simulink model "skarab_adc4x3g14_byp"  (R2018a)
settings: Solver=VariableStepAuto  StartTime=0.0  StopTime=10.0  RelTol=1e-3
libraries: xbsIndex_r4 x113
settings Model: Creator=aisaacson  LastModifiedBy=aisaacson

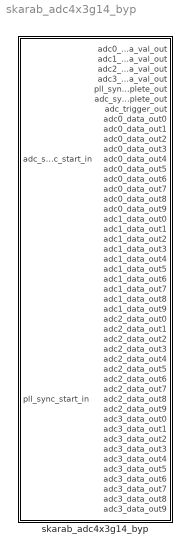
== system skarab_adc4x3g14_byp ==
  skarab_adc4x3g14_byp : Subsystem  Tag=xps:skarab_adc4x3g_14_byp  mask(hmc){mez=2}
      mask prompts: mez "Mezzanine slot"
      mask help: Interface to ADC cards available on SKARAB boards.
      mask init:
      | skarab_adc4x3g14_byp_mask(gcb);
      mask TypeOptions mez: 0 | 1 | 2 | 3
      mask DialogControl Container6 Prompt: Parameters

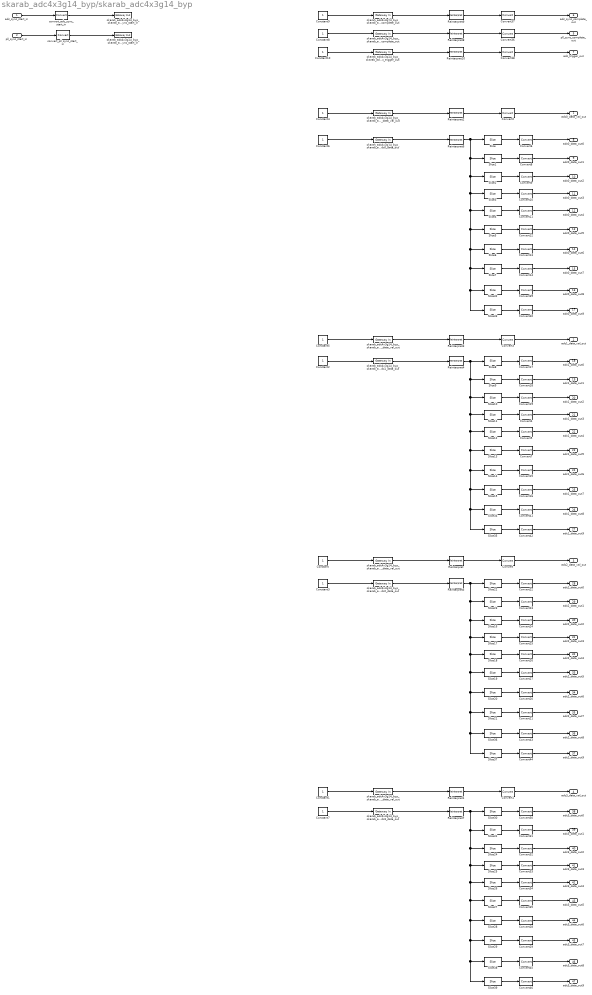
== system skarab_adc4x3g14_byp/skarab_adc4x3g14_byp ==
  adc_sync_start_in : Inport
  pll_sync_start_in : Inport  Port=2
  Constant{,1..10} (11 alike) : Constant
  Convert{,1..3,36..38} (7 alike) : xbsIndex_r4/Convert  gui_display_data_type=Boolean  arith_type=Boolean  n_bits=16  bin_pt=14  float_type=Single  exp_bits=8  fraction_bits=24  quantization=Truncate  overflow=Wrap  en=off  latency=0  pipeline=off  dbl_ovrd=off  block_type=convert
  Convert{4..35,39..46} (40 alike) : xbsIndex_r4/Convert  gui_display_data_type=Fixed-point  arith_type="Signed  (2's comp)"  n_bits=12  bin_pt=0  float_type=Single  exp_bits=8  fraction_bits=24  quantization=Truncate  overflow=Wrap  en=off  latency=0  pipeline=off  dbl_ovrd=off  block_type=convert
  Reinterpret{,1..10} (11 alike) : xbsIndex_r4/Reinterpret  force_arith_type=on  arith_type=Unsigned  force_bin_pt=on  bin_pt=0  block_type=reinterpret
  Slice{,8,22,30} (4 alike) : xbsIndex_r4/Slice  nbits=12  boolean_output=off  mode=Lower Bit Location + Width  bit1=0  base1=MSB of Input  bit0=0  base0=LSB of Input  dbl_ovrd=off  block_type=slice
  Slice{1,9,23,31} (4 alike) : xbsIndex_r4/Slice  nbits=12  boolean_output=off  mode=Lower Bit Location + Width  bit1=0  base1=MSB of Input  bit0=12  base0=LSB of Input  dbl_ovrd=off  block_type=slice
  Slice{2,10,16,24} (4 alike) : xbsIndex_r4/Slice  nbits=12  boolean_output=off  mode=Lower Bit Location + Width  bit1=0  base1=MSB of Input  bit0=24  base0=LSB of Input  dbl_ovrd=off  block_type=slice
  Slice{3,11,17,25} (4 alike) : xbsIndex_r4/Slice  nbits=12  boolean_output=off  mode=Lower Bit Location + Width  bit1=0  base1=MSB of Input  bit0=36  base0=LSB of Input  dbl_ovrd=off  block_type=slice
  Slice{4,12,18,26} (4 alike) : xbsIndex_r4/Slice  nbits=12  boolean_output=off  mode=Lower Bit Location + Width  bit1=0  base1=MSB of Input  bit0=48  base0=LSB of Input  dbl_ovrd=off  block_type=slice
  Slice{5,13,19,27} (4 alike) : xbsIndex_r4/Slice  nbits=12  boolean_output=off  mode=Lower Bit Location + Width  bit1=0  base1=MSB of Input  bit0=60  base0=LSB of Input  dbl_ovrd=off  block_type=slice
  Slice{6,14,20,28} (4 alike) : xbsIndex_r4/Slice  nbits=12  boolean_output=off  mode=Lower Bit Location + Width  bit1=0  base1=MSB of Input  bit0=72  base0=LSB of Input  dbl_ovrd=off  block_type=slice
  Slice{7,15,21,29} (4 alike) : xbsIndex_r4/Slice  nbits=12  boolean_output=off  mode=Lower Bit Location + Width  bit1=0  base1=MSB of Input  bit0=84  base0=LSB of Input  dbl_ovrd=off  block_type=slice
  Slice{32,34,36,38} (4 alike) : xbsIndex_r4/Slice  nbits=12  boolean_output=off  mode=Lower Bit Location + Width  bit1=0  base1=MSB of Input  bit0=96  base0=LSB of Input  dbl_ovrd=off  block_type=slice
  Slice{33,35,37,39} (4 alike) : xbsIndex_r4/Slice  nbits=12  boolean_output=off  mode=Lower Bit Location + Width  bit1=0  base1=MSB of Input  bit0=108  base0=LSB of Input  dbl_ovrd=off  block_type=slice
  convert_adc_sync_start_in : xbsIndex_r4/Convert  gui_display_data_type=Boolean  arith_type=Boolean  n_bits=16  bin_pt=14  float_type=Single  exp_bits=8  fraction_bits=24  quantization=Truncate  overflow=Wrap  en=off  latency=0  pipeline=off  dbl_ovrd=off  block_type=convert
  convert_pll_sync_start_in : xbsIndex_r4/Convert  gui_display_data_type=Boolean  arith_type=Boolean  n_bits=16  bin_pt=14  float_type=Single  exp_bits=8  fraction_bits=24  quantization=Truncate  overflow=Wrap  en=off  latency=0  pipeline=off  dbl_ovrd=off  block_type=convert
  skarab_adc4x3g14_byp_skarab_adc4x3g14_byp_adc0_data_out : xbsIndex_r4/Gateway In  gui_display_data_type=Fixed-point  arith_type=Unsigned  n_bits=128  bin_pt=0  preci_type=Single  exp_width=8  frac_width=24  rows=1  columns=1  quantization=Truncate  overflow=Wrap  period=1  UseAsADC=off  ADCChannel='1'  interface=None  automatic_assignment=on  address_offset=hex2dec('00')  intf_name=''  intf_description=''  default_value=0  timing_constraint=None  locs_specified=off  LOCs={}  io_standard={}  inherit_from_input=off  hdl_port=on  dbl_ovrd=off  block_type=gatewayin
  skarab_adc4x3g14_byp_skarab_adc4x3g14_byp_adc0_data_val_out : xbsIndex_r4/Gateway In  gui_display_data_type=Boolean  arith_type=Boolean  n_bits=16  bin_pt=14  preci_type=Single  exp_width=8  frac_width=24  rows=1  columns=1  quantization="Round  (unbiased: +/- Inf)"  overflow=Saturate  period=1  UseAsADC=off  ADCChannel='1'  interface=None  automatic_assignment=on  address_offset=hex2dec('00')  intf_name=''  intf_description=''  default_value=0  timing_constraint=None  locs_specified=off  LOCs={}  io_standard={}  inherit_from_input=off  hdl_port=on  dbl_ovrd=off  block_type=gatewayin
  skarab_adc4x3g14_byp_skarab_adc4x3g14_byp_adc1_data_out : xbsIndex_r4/Gateway In  gui_display_data_type=Fixed-point  arith_type=Unsigned  n_bits=128  bin_pt=0  preci_type=Single  exp_width=8  frac_width=24  rows=1  columns=1  quantization=Truncate  overflow=Wrap  period=1  UseAsADC=off  ADCChannel='1'  interface=None  automatic_assignment=on  address_offset=hex2dec('00')  intf_name=''  intf_description=''  default_value=0  timing_constraint=None  locs_specified=off  LOCs={}  io_standard={}  inherit_from_input=off  hdl_port=on  dbl_ovrd=off  block_type=gatewayin
  skarab_adc4x3g14_byp_skarab_adc4x3g14_byp_adc1_data_val_out : xbsIndex_r4/Gateway In  gui_display_data_type=Boolean  arith_type=Boolean  n_bits=16  bin_pt=14  preci_type=Single  exp_width=8  frac_width=24  rows=1  columns=1  quantization="Round  (unbiased: +/- Inf)"  overflow=Saturate  period=1  UseAsADC=off  ADCChannel='1'  interface=None  automatic_assignment=on  address_offset=hex2dec('00')  intf_name=''  intf_description=''  default_value=0  timing_constraint=None  locs_specified=off  LOCs={}  io_standard={}  inherit_from_input=off  hdl_port=on  dbl_ovrd=off  block_type=gatewayin
  skarab_adc4x3g14_byp_skarab_adc4x3g14_byp_adc2_data_out : xbsIndex_r4/Gateway In  gui_display_data_type=Fixed-point  arith_type=Unsigned  n_bits=128  bin_pt=0  preci_type=Single  exp_width=8  frac_width=24  rows=1  columns=1  quantization=Truncate  overflow=Wrap  period=1  UseAsADC=off  ADCChannel='1'  interface=None  automatic_assignment=on  address_offset=hex2dec('00')  intf_name=''  intf_description=''  default_value=0  timing_constraint=None  locs_specified=off  LOCs={}  io_standard={}  inherit_from_input=off  hdl_port=on  dbl_ovrd=off  block_type=gatewayin
  skarab_adc4x3g14_byp_skarab_adc4x3g14_byp_adc2_data_val_out : xbsIndex_r4/Gateway In  gui_display_data_type=Boolean  arith_type=Boolean  n_bits=16  bin_pt=14  preci_type=Single  exp_width=8  frac_width=24  rows=1  columns=1  quantization="Round  (unbiased: +/- Inf)"  overflow=Saturate  period=1  UseAsADC=off  ADCChannel='1'  interface=None  automatic_assignment=on  address_offset=hex2dec('00')  intf_name=''  intf_description=''  default_value=0  timing_constraint=None  locs_specified=off  LOCs={}  io_standard={}  inherit_from_input=off  hdl_port=on  dbl_ovrd=off  block_type=gatewayin
  skarab_adc4x3g14_byp_skarab_adc4x3g14_byp_adc3_data_out : xbsIndex_r4/Gateway In  gui_display_data_type=Fixed-point  arith_type=Unsigned  n_bits=128  bin_pt=0  preci_type=Single  exp_width=8  frac_width=24  rows=1  columns=1  quantization=Truncate  overflow=Wrap  period=1  UseAsADC=off  ADCChannel='1'  interface=None  automatic_assignment=on  address_offset=hex2dec('00')  intf_name=''  intf_description=''  default_value=0  timing_constraint=None  locs_specified=off  LOCs={}  io_standard={}  inherit_from_input=off  hdl_port=on  dbl_ovrd=off  block_type=gatewayin
  skarab_adc4x3g14_byp_skarab_adc4x3g14_byp_adc3_data_val_out : xbsIndex_r4/Gateway In  gui_display_data_type=Boolean  arith_type=Boolean  n_bits=16  bin_pt=14  preci_type=Single  exp_width=8  frac_width=24  rows=1  columns=1  quantization="Round  (unbiased: +/- Inf)"  overflow=Saturate  period=1  UseAsADC=off  ADCChannel='1'  interface=None  automatic_assignment=on  address_offset=hex2dec('00')  intf_name=''  intf_description=''  default_value=0  timing_constraint=None  locs_specified=off  LOCs={}  io_standard={}  inherit_from_input=off  hdl_port=on  dbl_ovrd=off  block_type=gatewayin
  skarab_adc4x3g14_byp_skarab_adc4x3g14_byp_adc_sync_complete_out : xbsIndex_r4/Gateway In  gui_display_data_type=Boolean  arith_type=Boolean  n_bits=16  bin_pt=14  preci_type=Single  exp_width=8  frac_width=24  rows=1  columns=1  quantization="Round  (unbiased: +/- Inf)"  overflow=Saturate  period=1  UseAsADC=off  ADCChannel='1'  interface=None  automatic_assignment=on  address_offset=hex2dec('00')  intf_name=''  intf_description=''  default_value=0  timing_constraint=None  locs_specified=off  LOCs={}  io_standard={}  inherit_from_input=off  hdl_port=on  dbl_ovrd=off  block_type=gatewayin
  skarab_adc4x3g14_byp_skarab_adc4x3g14_byp_adc_sync_start_in : xbsIndex_r4/Gateway Out  inherit_from_input=off  hdl_port=on  rows=1  columns=1  UseAsDAC=off  DACChannel='1'  interface=None  automatic_assignment=on  address_offset=hex2dec('00')  intf_name=''  intf_description=''  timing_constraint=None  locs_specified=off  LOCs={}  io_standard={}  block_type=gatewayout
  skarab_adc4x3g14_byp_skarab_adc4x3g14_byp_adc_trigger_out : xbsIndex_r4/Gateway In  gui_display_data_type=Boolean  arith_type=Boolean  n_bits=16  bin_pt=14  preci_type=Single  exp_width=8  frac_width=24  rows=1  columns=1  quantization="Round  (unbiased: +/- Inf)"  overflow=Saturate  period=1  UseAsADC=off  ADCChannel='1'  interface=None  automatic_assignment=on  address_offset=hex2dec('00')  intf_name=''  intf_description=''  default_value=0  timing_constraint=None  locs_specified=off  LOCs={}  io_standard={}  inherit_from_input=off  hdl_port=on  dbl_ovrd=off  block_type=gatewayin
  skarab_adc4x3g14_byp_skarab_adc4x3g14_byp_pll_sync_complete_out : xbsIndex_r4/Gateway In  gui_display_data_type=Boolean  arith_type=Boolean  n_bits=16  bin_pt=14  preci_type=Single  exp_width=8  frac_width=24  rows=1  columns=1  quantization="Round  (unbiased: +/- Inf)"  overflow=Saturate  period=1  UseAsADC=off  ADCChannel='1'  interface=None  automatic_assignment=on  address_offset=hex2dec('00')  intf_name=''  intf_description=''  default_value=0  timing_constraint=None  locs_specified=off  LOCs={}  io_standard={}  inherit_from_input=off  hdl_port=on  dbl_ovrd=off  block_type=gatewayin
  skarab_adc4x3g14_byp_skarab_adc4x3g14_byp_pll_sync_start_in : xbsIndex_r4/Gateway Out  inherit_from_input=off  hdl_port=on  rows=1  columns=1  UseAsDAC=off  DACChannel='1'  interface=None  automatic_assignment=on  address_offset=hex2dec('00')  intf_name=''  intf_description=''  timing_constraint=None  locs_specified=off  LOCs={}  io_standard={}  block_type=gatewayout
  adc0_data_val_out : Outport
  adc1_data_val_out : Outport  Port=2
  adc2_data_val_out : Outport  Port=3
  adc3_data_val_out : Outport  Port=4
  pll_sync_complete_out : Outport  Port=5
  adc_sync_complete_out : Outport  Port=6
  adc_trigger_out : Outport  Port=7
  adc0_data_out0 : Outport  Port=8
  adc0_data_out1 : Outport  Port=9
  adc0_data_out2 : Outport  Port=10
  adc0_data_out3 : Outport  Port=11
  adc0_data_out4 : Outport  Port=12
  adc0_data_out5 : Outport  Port=13
  adc0_data_out6 : Outport  Port=14
  adc0_data_out7 : Outport  Port=15
  adc0_data_out8 : Outport  Port=16
  adc0_data_out9 : Outport  Port=17
  adc1_data_out0 : Outport  Port=18
  adc1_data_out1 : Outport  Port=19
  adc1_data_out2 : Outport  Port=20
  adc1_data_out3 : Outport  Port=21
  adc1_data_out4 : Outport  Port=22
  adc1_data_out5 : Outport  Port=23
  adc1_data_out6 : Outport  Port=24
  adc1_data_out7 : Outport  Port=25
  adc1_data_out8 : Outport  Port=26
  adc1_data_out9 : Outport  Port=27
  adc2_data_out0 : Outport  Port=28
  adc2_data_out1 : Outport  Port=29
  adc2_data_out2 : Outport  Port=30
  adc2_data_out3 : Outport  Port=31
  adc2_data_out4 : Outport  Port=32
  adc2_data_out5 : Outport  Port=33
  adc2_data_out6 : Outport  Port=34
  adc2_data_out7 : Outport  Port=35
  adc2_data_out8 : Outport  Port=36
  adc2_data_out9 : Outport  Port=37
  adc3_data_out0 : Outport  Port=38
  adc3_data_out1 : Outport  Port=39
  adc3_data_out2 : Outport  Port=40
  adc3_data_out3 : Outport  Port=41
  adc3_data_out4 : Outport  Port=42
  adc3_data_out5 : Outport  Port=43
  adc3_data_out6 : Outport  Port=44
  adc3_data_out7 : Outport  Port=45
  adc3_data_out8 : Outport  Port=46
  adc3_data_out9 : Outport  Port=47
  wires:
  adc_sync_start_in/1 -> convert_adc_sync_start_in/1
  convert_adc_sync_start_in/1 -> skarab_adc4x3g14_byp_skarab_adc4x3g14_byp_adc_sync_start_in/1
  pll_sync_start_in/1 -> convert_pll_sync_start_in/1
  convert_pll_sync_start_in/1 -> skarab_adc4x3g14_byp_skarab_adc4x3g14_byp_pll_sync_start_in/1
  Constant/1 -> skarab_adc4x3g14_byp_skarab_adc4x3g14_byp_adc2_data_val_out/1
  skarab_adc4x3g14_byp_skarab_adc4x3g14_byp_adc2_data_val_out/1 -> Reinterpret/1
  Reinterpret/1 -> Convert/1
  Convert/1 -> adc2_data_val_out/1
  Constant1/1 -> skarab_adc4x3g14_byp_skarab_adc4x3g14_byp_adc3_data_val_out/1
  skarab_adc4x3g14_byp_skarab_adc4x3g14_byp_adc3_data_val_out/1 -> Reinterpret1/1
  Reinterpret1/1 -> Convert1/1
  Convert1/1 -> adc3_data_val_out/1
  Constant4/1 -> skarab_adc4x3g14_byp_skarab_adc4x3g14_byp_adc0_data_val_out/1
  skarab_adc4x3g14_byp_skarab_adc4x3g14_byp_adc0_data_val_out/1 -> Reinterpret2/1
  Reinterpret2/1 -> Convert2/1
  Convert2/1 -> adc0_data_val_out/1
  Constant5/1 -> skarab_adc4x3g14_byp_skarab_adc4x3g14_byp_adc1_data_val_out/1
  skarab_adc4x3g14_byp_skarab_adc4x3g14_byp_adc1_data_val_out/1 -> Reinterpret3/1
  Reinterpret3/1 -> Convert3/1
  Convert3/1 -> adc1_data_val_out/1
  Constant6/1 -> skarab_adc4x3g14_byp_skarab_adc4x3g14_byp_adc0_data_out/1
  skarab_adc4x3g14_byp_skarab_adc4x3g14_byp_adc0_data_out/1 -> Reinterpret6/1
  Reinterpret6/1 -> Slice33/1, Slice32/1, Slice7/1, Slice6/1, Slice5/1, Slice4/1, Slice3/1, Slice2/1, Slice1/1, Slice/1
  Convert6/1 -> adc0_data_out0/1
  Slice/1 -> Convert6/1
  Convert8/1 -> adc0_data_out1/1
  Slice1/1 -> Convert8/1
  Convert9/1 -> adc0_data_out2/1
  Slice2/1 -> Convert9/1
  Convert10/1 -> adc0_data_out3/1
  Slice3/1 -> Convert10/1
  Convert11/1 -> adc0_data_out4/1
  Slice4/1 -> Convert11/1
  Convert12/1 -> adc0_data_out5/1
  Slice5/1 -> Convert12/1
  Convert13/1 -> adc0_data_out6/1
  Slice6/1 -> Convert13/1
  Convert14/1 -> adc0_data_out7/1
  Slice7/1 -> Convert14/1
  Constant2/1 -> skarab_adc4x3g14_byp_skarab_adc4x3g14_byp_adc1_data_out/1
  skarab_adc4x3g14_byp_skarab_adc4x3g14_byp_adc1_data_out/1 -> Reinterpret4/1
  Reinterpret4/1 -> Slice34/1, Slice35/1, Slice15/1, Slice14/1, Slice13/1, Slice12/1, Slice11/1, Slice10/1, Slice9/1, Slice8/1
  Convert17/1 -> adc1_data_out0/1
  Slice8/1 -> Convert17/1
  Convert18/1 -> adc1_data_out1/1
  Slice9/1 -> Convert18/1
  Convert19/1 -> adc1_data_out2/1
  Slice10/1 -> Convert19/1
  Convert4/1 -> adc1_data_out3/1
  Slice11/1 -> Convert4/1
  Convert5/1 -> adc1_data_out4/1
  Slice12/1 -> Convert5/1
  Convert7/1 -> adc1_data_out5/1
  Slice13/1 -> Convert7/1
  Convert15/1 -> adc1_data_out6/1
  Slice14/1 -> Convert15/1
  Convert16/1 -> adc1_data_out7/1
  Slice15/1 -> Convert16/1
  Constant3/1 -> skarab_adc4x3g14_byp_skarab_adc4x3g14_byp_adc2_data_out/1
  skarab_adc4x3g14_byp_skarab_adc4x3g14_byp_adc2_data_out/1 -> Reinterpret5/1
  Reinterpret5/1 -> Slice37/1, Slice36/1, Slice21/1, Slice20/1, Slice19/1, Slice18/1, Slice17/1, Slice16/1, Slice23/1, Slice22/1
  Convert22/1 -> adc2_data_out0/1
  Slice22/1 -> Convert22/1
  Convert23/1 -> adc2_data_out1/1
  Slice23/1 -> Convert23/1
  Convert24/1 -> adc2_data_out2/1
  Slice16/1 -> Convert24/1
  Convert25/1 -> adc2_data_out3/1
  Slice17/1 -> Convert25/1
  Convert26/1 -> adc2_data_out4/1
  Slice18/1 -> Convert26/1
  Convert27/1 -> adc2_data_out5/1
  Slice19/1 -> Convert27/1
  Convert20/1 -> adc2_data_out6/1
  Slice20/1 -> Convert20/1
  Convert21/1 -> adc2_data_out7/1
  Slice21/1 -> Convert21/1
  Constant7/1 -> skarab_adc4x3g14_byp_skarab_adc4x3g14_byp_adc3_data_out/1
  skarab_adc4x3g14_byp_skarab_adc4x3g14_byp_adc3_data_out/1 -> Reinterpret7/1
  Reinterpret7/1 -> Slice39/1, Slice38/1, Slice29/1, Slice28/1, Slice27/1, Slice26/1, Slice25/1, Slice24/1, Slice31/1, Slice30/1
  Convert30/1 -> adc3_data_out0/1
  Slice30/1 -> Convert30/1
  Convert31/1 -> adc3_data_out1/1
  Slice31/1 -> Convert31/1
  Convert32/1 -> adc3_data_out2/1
  Slice24/1 -> Convert32/1
  Convert33/1 -> adc3_data_out3/1
  Slice25/1 -> Convert33/1
  Convert34/1 -> adc3_data_out4/1
  Slice26/1 -> Convert34/1
  Convert35/1 -> adc3_data_out5/1
  Slice27/1 -> Convert35/1
  Convert28/1 -> adc3_data_out6/1
  Slice28/1 -> Convert28/1
  Convert29/1 -> adc3_data_out7/1
  Slice29/1 -> Convert29/1
  Constant8/1 -> skarab_adc4x3g14_byp_skarab_adc4x3g14_byp_pll_sync_complete_out/1
  skarab_adc4x3g14_byp_skarab_adc4x3g14_byp_pll_sync_complete_out/1 -> Reinterpret8/1
  Reinterpret8/1 -> Convert36/1
  Convert36/1 -> pll_sync_complete_out/1
  Constant9/1 -> skarab_adc4x3g14_byp_skarab_adc4x3g14_byp_adc_sync_complete_out/1
  skarab_adc4x3g14_byp_skarab_adc4x3g14_byp_adc_sync_complete_out/1 -> Reinterpret9/1
  Reinterpret9/1 -> Convert37/1
  Convert37/1 -> adc_sync_complete_out/1
  Constant10/1 -> skarab_adc4x3g14_byp_skarab_adc4x3g14_byp_adc_trigger_out/1
  skarab_adc4x3g14_byp_skarab_adc4x3g14_byp_adc_trigger_out/1 -> Reinterpret10/1
  Reinterpret10/1 -> Convert38/1
  Convert38/1 -> adc_trigger_out/1
  Slice32/1 -> Convert39/1
  Slice33/1 -> Convert40/1
  Convert39/1 -> adc0_data_out8/1
  Convert40/1 -> adc0_data_out9/1
  Slice34/1 -> Convert41/1
  Convert41/1 -> adc1_data_out8/1
  Convert42/1 -> adc1_data_out9/1
  Slice35/1 -> Convert42/1
  Convert43/1 -> adc2_data_out8/1
  Convert44/1 -> adc2_data_out9/1
  Slice36/1 -> Convert43/1
  Slice37/1 -> Convert44/1
  Convert46/1 -> adc3_data_out9/1
  Convert45/1 -> adc3_data_out8/1
  Slice39/1 -> Convert46/1
  Slice38/1 -> Convert45/1
